simulink model "QBOT_follower1"  (R2022b)
settings: Solver=ode1  StartTime=0.0  StopTime=inf  FixedStep=Ts  RelTol=1e-3  EnableMultiTasking=on
model workspace (MAT data in the model file):
  Sig = Simulink.Signal
  Sig.DataType = 'auto'
  Sig.Dimensions = -1
  Sig.DimensionsMode = 'auto'
  Sig.Complexity = 'auto'
  Sig.SampleTime = -1
  Sig.SamplingMode = 'auto'
  downCamStepSize = Simulink.Parameter
  downCamStepSize.Value = Simulink.data.Expression
  downCamStepSize.Value.ExpressionString = "qc_get_step_size*ceil(1/60/qc_get_step_size)"
  downCamStepSize.DataType = 'auto'
  downCamStepSize.Complexity = 'real'
  downCamStepSize.Dimensions = -1
  lidarStepSize = Simulink.Parameter
  lidarStepSize.Value = Simulink.data.Expression
  lidarStepSize.Value.ExpressionString = "qc_get_step_size*ceil(1/5/qc_get_step_size)"
  lidarStepSize.DataType = 'auto'
  lidarStepSize.Complexity = 'real'
  lidarStepSize.Dimensions = -1
  mainStepSize = Simulink.Parameter
  mainStepSize.Value = Simulink.data.Expression
  mainStepSize.Value.ExpressionString = "qc_get_step_size"
  mainStepSize.DataType = 'auto'
  mainStepSize.Complexity = 'real'
  mainStepSize.Dimensions = -1
  mode = Simulink.Parameter
  mode.Value = 2
  mode.Description = '0 - education speeds via wheel speed commands
    | 1 - education speeds via body speed commands
    | 2 - research speeds via wheel speed commands
    | 3 - research speeds via body speed commands'
  mode.DataType = 'auto'
  mode.Complexity = 'real'
  mode.Dimensions = [1 1]
  realSenseStepSize = Simulink.Parameter
  realSenseStepSize.Value = Simulink.data.Expression
  realSenseStepSize.Value.ExpressionString = "qc_get_step_size*ceil(1/30/qc_get_step_size)"
  realSenseStepSize.DataType = 'auto'
  realSenseStepSize.Complexity = 'real'
  realSenseStepSize.Dimensions = -1
values from neighbouring files (symbols this model uses):
  b = 0.17    [follower_1_parameters.m]    (also in follower_2_parameters.m; leader_parameters.m)
  d = 0.393    [follower_1_parameters.m]    (also in follower_2_parameters.m; leader_parameters.m)
  d_safe = 0.75    [follower_1_parameters.m]    (also in follower_2_parameters.m = 0.8)
  delay1 = 4    [follower_1_parameters.m]
  parameters = [r d wrlmax Ts b]    [follower_1_parameters.m]    (also in follower_2_parameters.m; leader_parameters.m)
  Q_k = [Q_k Qi]    [follower_1_parameters.m]    (also in follower_2_parameters.m; leader_parameters.m)
  R = 0*eye(2)    [follower_1_parameters.m]    (also in follower_2_parameters.m; leader_parameters.m)
  r = 0.04445    [follower_1_parameters.m]    (also in follower_2_parameters.m; leader_parameters.m)
  R_d = 0*eye(2)    [follower_1_parameters.m]    (also in follower_2_parameters.m; leader_parameters.m)
  T = [[r/2 r/2];[r/d -r/d]]    [follower_1_parameters.m]    (also in follower_2_parameters.m; leader_parameters.m)
  Ts = 1/60    (= 0.0166666666667)    [follower_1_parameters.m]    (also in follower_2_parameters.m; leader_parameters.m)
  u_pre = [0;0]    [follower_1_parameters.m]    (also in follower_2_parameters.m; leader_parameters.m)
  X0 = [vicon_data(1); vicon_data(2); vicon_data(6)]    [follower_1_parameters.m]    (also in follower_2_parameters.m; leader_parameters.m)
libraries: quarc_library x13, simulink x5, spsDiscreteVariableTimeDelayLib x1, dspsigops x1
settings Model: SimulationMode=external  ExtModeTrigDuration=10000  Creator=mbohra  LastModifiedBy=user
settings SolverCC: AlgebraicLoopSolver=TrustRegion  PositivePriorityOrder=on
settings DataIOCC: ReturnWorkspaceOutputs=off
settings OptimizationCC: ReuseModelBlockBuffer=on
settings DebuggingCC: UnconnectedInputMsg=warning  UnconnectedOutputMsg=warning  UnconnectedLineMsg=warning  ArithmeticOperatorsInVariantConditions=warning
settings HardwareCC: ProdBitPerLong=64  ProdLargestAtomicInteger=LongLong  ProdLargestAtomicFloat=Double  ProdLongLongMode=on  ProdHWDeviceType=ARM Compatible->ARM 64-bit (LP64)
settings ModelReferenceCC: EnableRefExpFcnMdlSchedulingChecks=on
settings SFSimCC: SimUseLocalCustomCode=off  CustomCodeUndefinedFunction=UseInterfaceOnly
settings RTWCC: Description=QUARC Linux QBot Platform Target Using Toolchain  SystemTargetFile=quarc_linux_qbot_platform.tlc  TemplateMakefile=quarc_default_tmf  RTWUseLocalCustomCode=off  Toolchain=QUARC linux_qbot_platform | gmake (64-bit Windows)  BuildConfiguration=Faster Runs
settings CodeAppCC: StateflowObjectComments=on
settings STFCustomTargetCC: TargetLangStandard=C99 (ISO)  ConcurrentExecutionCompliant=on  GRTInterface=on  UseToolchainInfoCompliant=on  SystemTargetFile=quarc_linux_qbot_platform.tlc
settings GRTTargetCC: ParMdlRefBuildCompliant=off  CompOptLevelCompliant=off  CombineOutputUpdateFcns=off  MatFileLogging=off  CPPClassGenCompliant=off  GRTInterface=on  ExtMode=on  ExtModeMexFile=quarc_comm  ExtModeMexArgs='-w -d /tmp -uri %u','tcpip://192.168.0.130:17001'
settings ConfigComp: CovMetricSettings=dswe

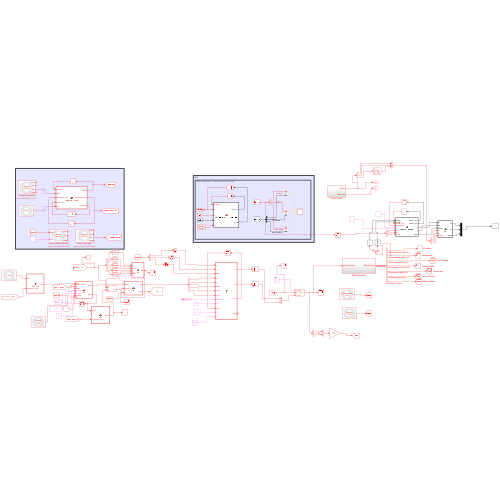
[thumbnail: Simulink's stored preview of the top-level diagram]
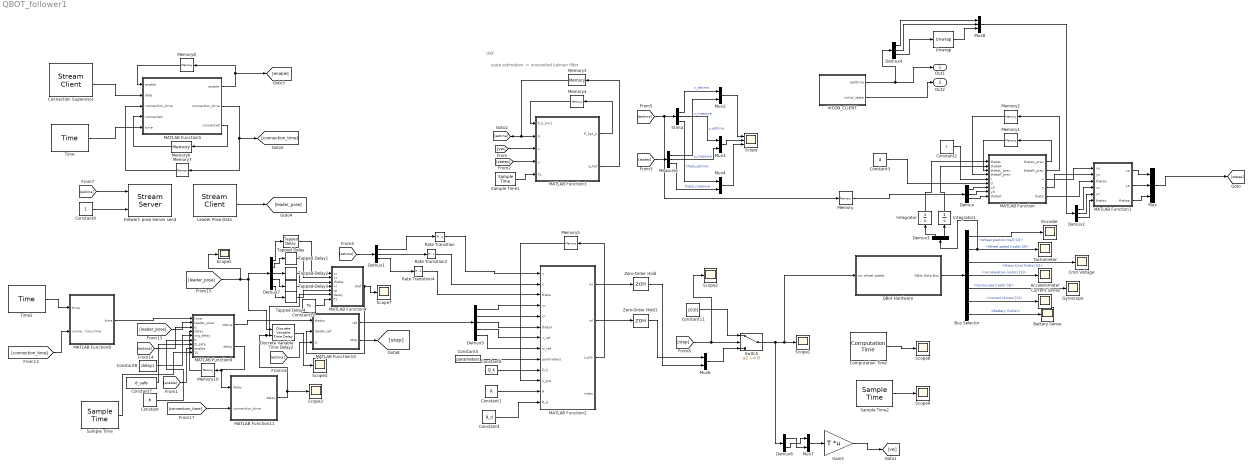
== system QBOT_follower1 ==
  note: UKF
  note: state estimation -> unscented kalman filter
  Accelerometer : Scope
  Battery Sense : Scope
  Bus Selector : BusSelector  OutputSignals=Wheel position (rad) [2],Wheel speed (rad/s) [2],Motor Cmd (Volts) [2],Acceleration (m/s/s) [3],Gyroscope (rad/s) [3],Current (Amps) [2],Battery (Volts)
  Cmd Voltage : Scope
  Computation Time : quarc_library/Sources/Time/Computation Time  sample_time=qc_get_step_size  use_model=on  use_cpu_time=off
  Connection Supervisor : quarc_library/Communications/Basic/Stream Client  uri_source=Specify via dialog (do not evaluate)  uri=tcpip://192.168.0.5:18013  send_buffer_size=1460  receive_buffer_size=1460  byte_order=little endian (Intel - LSB first)  optimization=Minimum latency  send_options=Do not send data  receive_options=Receive all data  default_value=[0]  sample_time=-1  active=off  implementation=Use blocking I/O in a separate thread  send_fifo_size=1000  receive_fifo_size=1000  send_priority=0  receive_priority=0  send_dimensions=off  receive_dimensions=off  max_dimensions=-1  data_type=Inherited via back propagation  type_expr=BusObject
      settings: AttributesFormatString="\"tcpip://192.168.0.5:18013\""
  Constant : Constant  Value=b
  Constant1 : Constant  Value=R
  Constant10 : Constant  Value=Ts
  Constant11 : Constant  Value=[0;0]  VectorParams1D=off
  Constant2 : Constant  Value=r
  Constant3 : Constant  Value=d
  Constant4 : Constant  Value=R_d
  Constant5 : Constant  Value=parameters
  Constant6 : Constant  Value=Q_k
  Constant7 : Constant  Value=d_safe
  Constant8 : Constant  Value=delay1
  Constant9 : Constant
  Current Sense : Scope
  Demux{,1..2,4} (4 alike) : Demux  Outputs=3
  Demux3 : Demux  Outputs=2
  Demux5 : Demux  Outputs=5
  Demux6 : Demux  Outputs=2
  Demux7 : Demux  Outputs=5
  Discrete Variable Time Delay2 : spsDiscreteVariableTimeDelayLib/Discrete Variable Time Delay  MaxDelay=60  InitialValue=0  Ts=Ts  DFT=on
      settings: LibrarySourceBlock=|
      | sps_lib/Control/Discrete Variable
      | Time Delay
  Encoder : Scope
  Follwer1 pose Server send : quarc_library/Communications/Basic/Stream Server  uri_source=Specify via dialog (do not evaluate)  uri=tcpip://192.168.0.130:18012  send_buffer_size=1460  receive_buffer_size=1460  byte_order=little endian (Intel - LSB first)  optimization=Minimum latency  send_options=Send all data  receive_options=Do not receive data  default_value=[0]  sample_time=-1  active=off  implementation=Use blocking I/O in a separate thread  send_fifo_size=1000  receive_fifo_size=1000  send_priority=0  receive_priority=0  send_dimensions=off  receive_dimensions=off  max_dimensions=-1  data_type=Inherited via back propagation  type_expr=BusObject
      settings: AttributesFormatString="\"tcpip://192.168.0.130:18012\""
  Gain5 : Gain  Gain=T  Multiplication=Matrix(K*u)
  Gyroscope : Scope
  Integrator : Integrator
  Integrator1 : Integrator
  Leader Pose Data : quarc_library/Communications/Basic/Stream Client  uri_source=Specify via dialog (do not evaluate)  uri=tcpip://192.168.0.230:18010  send_buffer_size=1460  receive_buffer_size=1460  byte_order=little endian (Intel - LSB first)  optimization=Minimum latency  send_options=Do not send data  receive_options=Receive all data  default_value=[0;0;0;0;0]  sample_time=-1  active=off  implementation=Use blocking I/O in a separate thread  send_fifo_size=1000  receive_fifo_size=1000  send_priority=0  receive_priority=0  send_dimensions=off  receive_dimensions=off  max_dimensions=-1  data_type=Inherited via back propagation  type_expr=BusObject
      settings: AttributesFormatString="\"tcpip://192.168.0.230:18010\""
  MATLAB Function : MATLAB Function  TreatAsAtomicUnit=on
  MATLAB Function1 : MATLAB Function  TreatAsAtomicUnit=on
  MATLAB Function10 : MATLAB Function  TreatAsAtomicUnit=on
  MATLAB Function11 : MATLAB Function  TreatAsAtomicUnit=on
  MATLAB Function2 : MATLAB Function  TreatAsAtomicUnit=on
  MATLAB Function3 : MATLAB Function  TreatAsAtomicUnit=on
  MATLAB Function4 : MATLAB Function  TreatAsAtomicUnit=on
  MATLAB Function5 : MATLAB Function  TreatAsAtomicUnit=on
  MATLAB Function8 : MATLAB Function  TreatAsAtomicUnit=on
  MATLAB Function9 : MATLAB Function  TreatAsAtomicUnit=on
  Measures : Demux  Outputs=3
  Memory : Memory  InitialCondition=X0
  Memory{1..2,6..8} (5 alike) : Memory
  Memory10 : Memory  InitialCondition=delay1
  Memory3 : Memory  InitialCondition=X0  InheritSampleTime=on
  Memory4 : Memory  InitialCondition=1e-6*eye(3)  InheritSampleTime=on
  Memory5 : Memory  InitialCondition=u_pre
  Mux : Mux  Inputs=3
  Mux{2..4,6..7} (5 alike) : Mux  Inputs=2
  Mux8 : Mux  Inputs=3
  QBot Hardware : Subsystem
  Rate Transition : RateTransition  OutPortSampleTime=Ts
  Rate Transition2 : RateTransition  OutPortSampleTime=Ts
  Rate Transition4 : RateTransition  OutPortSampleTime=Ts
  Sample Time : quarc_library/Sources/Time/Sample Time  Priority=-99  sample_time=qc_get_step_size
  Sample Time1 : quarc_library/Sources/Time/Sample Time  Priority=-99  sample_time=Ts
  Sample Time2 : quarc_library/Sources/Time/Sample Time  Priority=-99  sample_time=qc_get_step_size
  Scope : Scope  NumInputPorts=3
  Scope{1..8} (8 alike) : Scope
  Stima : Demux  Outputs=3
  Switch : Switch  Criteria=u2 ~= 0  SaturateOnIntegerOverflow=off  InputSameDT=off
  Tachometer : Scope
  Tapped Delay{,1..4} (5 alike) : simulink/Discrete/Tapped Delay  vinit=0.0  samptime=Ts  NumDelays=1500  DelayOrder=Newest  includeCurrent=on
  Time : quarc_library/Sources/Time/Time  time_source=Wall clock  sample_time=qc_get_step_size
  Time2 : quarc_library/Sources/Time/Time  time_source=Wall clock  sample_time=qc_get_step_size
  Unwrap : dspsigops/Unwrap  tol=pi  InputProcessing=Columns as channels (frame based)  running=off
  VICON_CLIENT : Subsystem
  Zero-Order Hold : ZeroOrderHold  SampleTime=Ts
  Zero-Order Hold1 : ZeroOrderHold  SampleTime=Ts
  Out1 : Outport
  Out2 : Outport  Port=2
  wires:
  QBot Hardware/1(QBot Data Bus) -> Bus Selector/1
  Bus Selector/1 -> Encoder/1  "<Wheel position (rad) [2]>"
  Bus Selector/3 -> Cmd Voltage/1  "<Motor Cmd (Volts) [2]>"
  Bus Selector/4 -> Accelerometer/1  "<Acceleration (m/s/s) [3]>"
  Bus Selector/6 -> Current Sense/1  "<Current (Amps) [2]>"
  Bus Selector/2 -> Demux3/1, Tachometer/1  "<Wheel speed (rad/s) [2]>"
  Bus Selector/5 -> Gyroscope/1  "<Gyroscope (rad/s) [3]>"
  Bus Selector/7 -> Battery Sense/1  "<Battery (Volts)>"
  VICON_CLIENT/1(realtime) -> Demux4/1, Out1/1
  VICON_CLIENT/2(initial_state) -> Out2/1
  MATLAB Function/3(x) -> MATLAB Function1/1(xo)
  MATLAB Function/4(y) -> MATLAB Function1/2(yo)
  MATLAB Function/5(theta) -> MATLAB Function1/3(thetao)
  Demux2/1 -> MATLAB Function1/4(xv)
  Demux2/2 -> MATLAB Function1/5(yv)
  Demux2/3 -> MATLAB Function1/6(thetav)
  MATLAB Function1/1(xa) -> Mux/1
  MATLAB Function1/2(ya) -> Mux/2
  MATLAB Function1/3(thetaa) -> Mux/3
  Mux/1 -> [states]
  Stima/1 -> Mux2/1  "x_estima"
  Sample Time1/1 -> MATLAB Function3/5(Ts)
  Measures/2 -> Mux3/2  "y_measure"
  Memory4/1 -> MATLAB Function3/1(P_k_km1)
  Measures/1 -> Mux2/2  "x_measure"
  Mux2/1 -> Scope/1
  [vw] -> MATLAB Function3/3(u)
  Mux3/1 -> Scope/2
  [states] -> Measures/1
  Stima/2 -> Mux3/1  "y_estima"
  Measures/3 -> Mux4/2  "theta_measure"
  [states] -> MATLAB Function3/4(y)
  [estima] -> Memory/1, Stima/1
  MATLAB Function3/2(q_hat) -> Memory3/1
  Memory3/1 -> MATLAB Function3/2(q), [estima]
  Mux4/1 -> Scope/3
  MATLAB Function3/1(P_kp1_k) -> Memory4/1
  Stima/3 -> Mux4/1  "theta_estima"
  Constant3/1 -> MATLAB Function/6(d)
  Demux3/1 -> Integrator/1
  Demux3/2 -> Integrator1/1
  Integrator/1 -> MATLAB Function/1(thetaL)
  Integrator1/1 -> MATLAB Function/2(thetaR)
  Demux/3 -> MATLAB Function/9(theta0)
  Demux/1 -> MATLAB Function/7(x0)
  Demux/2 -> MATLAB Function/8(y0)
  Memory/1 -> Demux/1
  Constant2/1 -> MATLAB Function/5(r)
  MATLAB Function/1(thetaL_prev) -> Memory1/1
  MATLAB Function/2(thetaR_prev) -> Memory2/1
  Memory1/1 -> MATLAB Function/3("thetaL_prev ")
  Memory2/1 -> MATLAB Function/4("thetaR_prev ")
  Demux1/2 -> Rate Transition2/1
  Demux1/1 -> Rate Transition/1
  Rate Transition4/1 -> MATLAB Function2/3(theta)
  Constant6/1 -> MATLAB Function2/10(Q_k)
  Zero-Order Hold/1 -> Mux6/2
  MATLAB Function2/2(wl) -> Zero-Order Hold1/1
  Memory5/1 -> MATLAB Function2/11("u_pre ")
  Demux1/3 -> Rate Transition4/1
  Rate Transition/1 -> MATLAB Function2/1(x)
  Rate Transition2/1 -> MATLAB Function2/2(y)
  MATLAB Function2/1(wr) -> Zero-Order Hold/1
  Constant5/1 -> MATLAB Function2/9(parameters)
  MATLAB Function2/3(u_pre) -> Memory5/1
  Zero-Order Hold1/1 -> Mux6/1
  Constant4/1 -> MATLAB Function2/13(R_d)
  [estima] -> Demux1/1
  Constant1/1 -> MATLAB Function2/12(R)
  Gain5/1 -> [vw]
  Demux4/3 -> Unwrap/1
  Unwrap/1 -> Mux8/3
  Demux4/1 -> Mux8/1
  Demux4/2 -> Mux8/2
  Mux8/1 -> Demux2/1
  Demux5/1 -> MATLAB Function2/4(xr)
  Demux5/2 -> MATLAB Function2/5(yr)
  Demux5/3 -> MATLAB Function2/6(thetar)
  Demux5/4 -> MATLAB Function2/7(v_ref)
  Demux5/5 -> MATLAB Function2/8(w_ref)
  Constant11/1 -> Switch/1
  [stop] -> Scope2/1, Switch/2
  Mux6/1 -> Switch/3
  Switch/1 -> Demux6/1, QBot Hardware/1(rsc wheel speed), Scope1/1
  Demux6/1 -> Mux7/2
  Demux6/2 -> Mux7/1
  Mux7/1 -> Gain5/1
  Connection Supervisor/3 -> MATLAB Function5/2(data)
  MATLAB Function5/1(enable) -> Memory8/1, [enable]
  [estima] -> Follwer1 pose Server send/1
  Leader Pose Data/3 -> [leader_pose]
  MATLAB Function5/3(connected) -> Memory6/1
  Memory6/1 -> MATLAB Function5/4("connected ")
  Time/1 -> MATLAB Function5/5(time)
  MATLAB Function5/2(connection_time) -> Memory7/1, [connection_time]
  Memory7/1 -> MATLAB Function5/3("connection_time ")
  Memory8/1 -> MATLAB Function5/1("enable ")
  Time2/1 -> MATLAB Function8/1("time ")
  [connection_time] -> MATLAB Function8/2(connection_time)
  [leader_pose] -> MATLAB Function9/2(leader_pose)
  MATLAB Function8/1(time) -> MATLAB Function9/1(time)
  [estima] -> MATLAB Function9/3(q)
  MATLAB Function9/2(delay) -> MATLAB Function11/1("delay "), Memory10/1
  Memory10/1 -> MATLAB Function9/4("delay ")
  Constant8/1 -> MATLAB Function9/5(org_delay)
  MATLAB Function9/1(status) -> MATLAB Function10/1(status)
  Discrete Variable Time Delay2/1 -> Scope4/1
  [leader_pose] -> Scope5/1, Demux7/1, Discrete Variable Time Delay2/1
  [estima] -> MATLAB Function10/3(q)
  [connection_time] -> MATLAB Function11/2(connection_time)
  MATLAB Function11/1(delay) -> Scope3/1, MATLAB Function4/6(delay), Discrete Variable Time Delay2/2
  MATLAB Function10/1(ref) -> Demux5/1
  MATLAB Function10/2(stop) -> [stop]
  Constant/1 -> MATLAB Function9/6(b)
  Constant7/1 -> MATLAB Function9/7(D_safe)
  Constant9/1 -> Follwer1 pose Server send/2
  [enable] -> MATLAB Function9/8(enable)
  Sample Time/1 -> MATLAB Function9/9(Ts)
  Sample Time2/1 -> Scope6/1
  Demux7/4 -> Tapped Delay3/1
  Tapped Delay3/1 -> MATLAB Function4/4(vr)
  Tapped Delay1/1 -> MATLAB Function4/2(yr)
  Tapped Delay4/1 -> MATLAB Function4/5(wr)
  Tapped Delay/1 -> MATLAB Function4/1(xr)
  Tapped Delay2/1 -> MATLAB Function4/3(thetar)
  Demux7/1 -> Tapped Delay/1
  Demux7/5 -> Tapped Delay4/1
  Demux7/3 -> Tapped Delay2/1
  Demux7/2 -> Tapped Delay1/1
  Constant10/1 -> MATLAB Function4/7(Ts)
  MATLAB Function4/1(dref) -> MATLAB Function10/2(leader_ref), Scope7/1
  Computation Time/1 -> Scope8/1

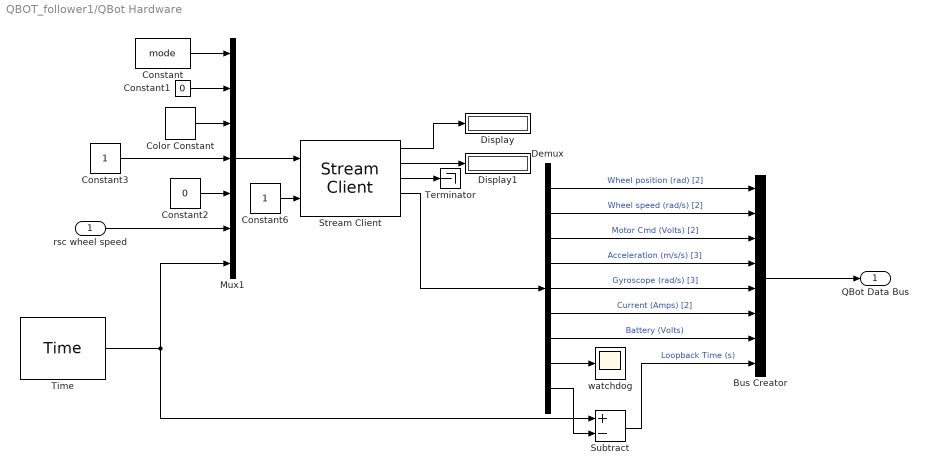
== system QBOT_follower1/QBot Hardware ==
  rsc wheel speed : Inport
  Bus Creator : BusCreator  Inputs=8
  Color Constant : quarc_library/Sources/Signals/Color Constant  color=[0 1 1]
      settings: SourceProductName=QUARC Targets
  Constant : Constant  Value=mode
  Constant1 : Constant  Value=0
  Constant2 : Constant  Value=0
  Constant3 : Constant
  Constant6 : Constant
  Demux : Demux  Outputs=[2 2 2 3 3 2 1 1 1]
  Display : Display
  Display1 : Display
  Mux1 : Mux  Inputs=7
  Stream Client : quarc_library/Communications/Basic/Stream Client  uri_source=Specify via dialog (do not evaluate)  uri=tcpip://localhost:18888  send_buffer_size=1460  receive_buffer_size=1460  byte_order=little endian (Intel - LSB first)  optimization=Minimum latency  send_options=Send most recent data  receive_options=Receive most recent data  default_value=zeros(17,1)  sample_time=qc_get_step_size  active=off  implementation=Use blocking I/O in a separate thread  send_fifo_size=1000  receive_fifo_size=1000  send_priority=0  receive_priority=0  send_dimensions=off  receive_dimensions=off  max_dimensions=-1  data_type=Inherited via back propagation  type_expr=BusObject
      settings: AttributesFormatString="\"tcpip://localhost:18888\""
  Subtract : Sum  Inputs=+-
  Terminator : Terminator
  Time : quarc_library/Sources/Time/Time  time_source=Wall clock  sample_time=qc_get_step_size
  watchdog : Scope
  QBot Data Bus : Outport
  wires:
  Demux/2 -> Bus Creator/2  "Wheel speed (rad/s) [2]"
  Constant/1 -> Mux1/1
  Stream Client/3 -> Terminator/1
  Stream Client/1 -> Display/1
  Constant6/1 -> Stream Client/2
  Stream Client/2 -> Display1/1
  Color Constant/1 -> Mux1/3
  Constant1/1 -> Mux1/2
  Demux/3 -> Bus Creator/3  "Motor Cmd (Volts) [2]"
  Mux1/1 -> Stream Client/1
  Stream Client/4 -> Demux/1
  Demux/1 -> Bus Creator/1  "Wheel position (rad) [2]"
  Demux/7 -> Bus Creator/7  "Battery (Volts)"
  Demux/5 -> Bus Creator/5  "Gyroscope (rad/s) [3]"
  Demux/6 -> Bus Creator/6  "Current (Amps) [2]"
  Demux/9 -> Subtract/2
  Constant2/1 -> Mux1/5
  Demux/4 -> Bus Creator/4  "Acceleration (m/s/s) [3]"
  Time/1 -> Subtract/1, Mux1/7
  Bus Creator/1 -> QBot Data Bus/1
  Subtract/1 -> Bus Creator/8  "Loopback Time (s)"
  Demux/8 -> watchdog/1
  Constant3/1 -> Mux1/4
  rsc wheel speed/1 -> Mux1/6

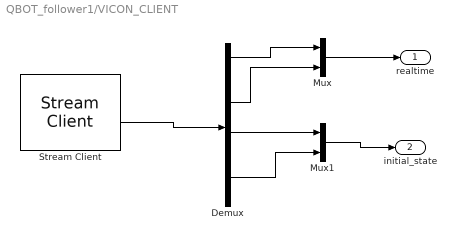
== system QBOT_follower1/VICON_CLIENT ==
  Demux : Demux  Outputs=[2 1 2 1 1 2 1 2 1 1]
  Mux : Mux  Inputs=2
  Mux1 : Mux  Inputs=2
  Stream Client : quarc_library/Communications/Basic/Stream Client  uri_source=Specify via dialog (do not evaluate)  uri=tcpip://192.168.0.5:18099  send_buffer_size=1460  receive_buffer_size=1460  byte_order=little endian (Intel - LSB first)  optimization=Minimum latency  send_options=Do not send data  receive_options=Receive most recent data  default_value=zeros(1,14)  sample_time=-1  active=off  implementation=Use blocking I/O in a separate thread  send_fifo_size=1000  receive_fifo_size=1000  send_priority=0  receive_priority=0  send_dimensions=off  receive_dimensions=off  max_dimensions=-1  data_type=Inherited via back propagation  type_expr=BusObject
      settings: AttributesFormatString="\"tcpip://192.168.0.5:18099\""
  realtime : Outport
  initial_state : Outport  Port=2
  wires:
  Stream Client/3 -> Demux/1
  Demux/9 -> Mux1/2
  Demux/4 -> Mux/2
  Demux/6 -> Mux1/1
  Demux/1 -> Mux/1
  Mux1/1 -> initial_state/1
  Mux/1 -> realtime/1

== matlab function QBOT_follower1/MATLAB Function8 ==
  data: time input; time output; connection_time input
function time = time_chn(time, connection_time)

time = time - connection_time

== matlab function QBOT_follower1/MATLAB Function9 ==
  data: status output; time input; delay output; leader_pose input; q input; delay input; org_delay input; b input; D_safe input; enable input; Ts input
function [status,delay]= fcn(time, leader_pose, q, delay, org_delay,b, D_safe, enable,Ts)

leader_B=[leader_pose(1)+b*cos(leader_pose(3));leader_pose(2)+b*sin(leader_pose(3))];
follower1_B=[q(1)+b*cos(q(3));q(2)+b*sin(q(3))];

% leader_B=[leader_pose(1);leader_pose(2)];
% follower1_B=[q(1);q(2)];


%stop = 1, Go = 0
if time<delay
    status = 1;
else
   
    if check_intersection(leader_B,follower1_B,D_safe)
        status = 1;
        delay = delay+Ts;
    else
        if delay>org_delay
            delay = delay-Ts;
        end
        status = 0;
    end
end

if enable == 0
    status = 1;
end

end

function collision = check_intersection(z1,z2,d_safe)
if  norm(z1-z2,2)<d_safe %||  norm(z1-z2,2)<r1+r2
    collision=1;
else
    collision=0;
end

end

== matlab function QBOT_follower1/MATLAB Function10 ==
  data: status input; ref output; leader_ref input; q input; stop output
function [ref, stop]= fcn(status,leader_ref, q)

if status == 1
    stop =1;
    ref = [q;0;0];
else
    stop =0;
    ref = leader_ref;
end

== matlab function QBOT_follower1/MATLAB Function2 ==
  data: x input; wr output; y input; theta input; xr input; yr input; wl output; thetar input; v_ref input; w_ref input; parameters input; Q_k input; u_pre input; u_pre output; R input; R_d input; index output
function [wr, wl, u_pre,index] = fcn(x,y,theta,xr,yr,thetar,v_ref,w_ref, parameters, Q_k,u_pre, R,R_d)

r=parameters(1);        % radius od wheels [m]
d=parameters(2);      % distance between the two wheels [m]
wrlmax=parameters(3);   % max angular velocity [rad/s] 
Ts=parameters(4);      % sampling time [s]
b=parameters(5);         % distance point b [m]


T=[[r/2 r/2];[r/d -r/d]];
T_inv=inv(T);
Hd=[-1/wrlmax 0 ; 0 -1/wrlmax ; 1/wrlmax 0 ; 0 1/wrlmax];


A = eye(2);
Bu = eye(2)*Ts;
Bd = eye(2)*Ts;


z_curr=[x+b*cos(theta)-(xr+b*cos(thetar));
        y+b*sin(theta)-(yr+b*sin(thetar))];
    
    
    
    T_FL = [cos(theta) sin(theta); -sin(theta)/b cos(theta)/b];
    T_FL_inv=inv(T_FL);
    
    %Compute current input constraint set
    %     U_curr=T_FL_inv*U_uni;
    
    H_curr=Hd*T_inv*T_FL;
    g=ones(4,1);
    % U_curr=Polyhedron(H_curr,g);
    


    Qpre=Q_k(1:2,1:2); %DOUBLE CHECK%%%%%%%%%%%%%%%%%%%%%%%%%%%%%%%%%%%%%%%%
    index=inf;

    isintern=0;
    for j=1:2:length(Q_k)
        Q_curr=Q_k(1:2,j:j+1);
        if  z_curr'*inv(Q_curr)*z_curr<=1
            
            index=(j-1)/2+1;
            isintern=1;
            if index>1
                Qpre=Q_k(1:2,j-2:j-1);
            end
            break
        end
    end
    
    
    
    if isintern==0
        error('The current point is outside the domain of attraction of the algorithm')
    end
    
    
    
    T_FL_r=[cos(thetar) sin(thetar); -sin(thetar)/b cos(thetar)/b];
    ur=inv(T_FL_r)*[v_ref;w_ref];
   

    
    if index>1
        
  
        ukhat = online_phase_CDC(z_curr,Qpre,A,Bu,H_curr,g,R_d,ur,u_pre);
     
        
       
    else
        
        ukhat=-inv(Bd)*z_curr;
        
        ur=online_terminal_optim_QP(ur,ukhat,H_curr,g);

    end
    
    
    uk=ukhat+ur;
    u_pre=ukhat;
    
 
    
    
    
    vw=T_FL*uk;
    
    wrwl=T_inv*vw;


    wr=wrwl(1);
    wl=wrwl(2);




end





function uk = online_phase_CDC(x_curr,Qpre,A,B,H,g,Rd,ur,u_pre)



%Set theoretic MPC online optimization
obj_fun=@(u)(A*x_curr+B*(u+ur)-B*ur)'*(A*x_curr+B*(u+ur)-B*ur)+(u-u_pre)'*Rd*(u-u_pre);


    function [c,ceq]=quad_constr(u,H,g,Qpre,ur,A,B,x_curr)
        c1=H*(u+ur)-g;
        c2=(A*x_curr+B*(u+ur)-B*ur)'*inv(Qpre)*(A*x_curr+B*(u+ur)-B*ur)-1;
        c=[c1;c2];
        ceq=[];
    end



options=optimoptions('fmincon','Display','off','Algorithm','sqp');
usol = fmincon(obj_fun,[0;0],[],[],[],[],[],[],@(u)quad_constr(u,H,g,Qpre,ur,A,B,x_curr),options);
uk=usol;


test_g=H*(uk+ur)-g;

test1=test_g(1);
test2=test_g(2);
test3=test_g(3);
test4=test_g(4);

test5=(A*x_curr+B*(uk))'*inv(Qpre)*(A*x_curr+B*(uk))-1;


test=test1<0 & test2<0 & test3<0 &test4<0 & test5<0;


obj_fun=(A*x_curr+B*(uk+ur)-B*ur)'*(A*x_curr+B*(uk+ur)-B*ur)+(uk-u_pre)'*Rd*(uk-u_pre);




% if test~=1
% 
%     error('ATTENZIONE')
% 
% end



end




function ur_hat = online_terminal_optim_QP(ur,u0,H,g)


H_obj=eye(2);
f_obj=-ur;
A_constr=H;
b_constr=g-H*u0;


options = optimoptions(@quadprog,'Algorithm','active-set','Display','off');


usol=quadprog(H_obj,f_obj,A_constr,b_constr,[],[],[],[],[0;0],options);
ur_hat=usol;

end

== matlab function QBOT_follower1/MATLAB Function11 ==
  data: delay input; connection_time input; delay output
function delay = fcn(delay,connection_time)

delay = delay; %+ connection_time;

end

== matlab function QBOT_follower1/MATLAB Function1 ==
  data: xo input; xa output; yo input; thetao input; xv input; yv input; thetav input; ya output; thetaa output
function [xa,ya,thetaa] = fcn(xo,yo,thetao,xv,yv,thetav)
% a - average
% v- vicon_data
% o - odometry
 mo = 5;
 mv = 95;

xa = (mo*xo+mv*xv)/100;
ya = (mo*yo+mv*yv)/100;
thetaa = (mo*thetao+mv*thetav)/100;

== matlab function QBOT_follower1/MATLAB Function ==
  data: thetaL_prev output; thetaR_prev output; x output; thetaL input; y output; thetaR input; thetaL_prev input; thetaR_prev input; r input; d input; x0 input; y0 input; theta0 input; theta output
function [thetaL_prev, thetaR_prev,x,y,theta]=computeOdometry(thetaL,thetaR,thetaL_prev, thetaR_prev,r,d,x0,y0,theta0)
    delta_sL=r*(thetaL - thetaL_prev);
    delta_sR=r*(thetaR - thetaR_prev);
    delta_theta=(delta_sR-delta_sL)/d;
    delta_s=(delta_sR+delta_sL)/2;
    theta=theta0+delta_theta/2;
    x=x0+delta_s*cos(theta);
    y=y0+delta_s*sin(theta); 
    thetaL_prev = thetaL;
    thetaR_prev = thetaR;
end

== matlab function QBOT_follower1/MATLAB Function4 ==
  data: xr input; yr input; thetar input; vr input; wr input; dref output; delay input; Ts input
function dref = fcn(xr, yr, thetar, vr, wr, delay,Ts)
n = delay/Ts;
xrn = xr(n+1);
yrn = yr(n+1);
thetarn = thetar(n+1);
vrn = vr(n+1);
wrn = wr(n+1);
dref= [xrn;yrn;thetarn; vrn; wrn];
end

== matlab function QBOT_follower1/MATLAB Function5 ==
  data: enable input; data input; enable output; connection_time input; connection_time output; connected input; connected output; time input
function [enable,connection_time,connected] = resetconnection( enable,data,connection_time,connected, time)


if connected == 0
    connection_time = time;
    if data ==1
        connected = 1;
        enable = 1 ;
    end
end

== matlab function QBOT_follower1/MATLAB Function3 ==
  data: P_k_km1 input; P_kp1_k output; q input; u input; q_hat output; y input; Ts input
function [P_kp1_k,q_hat]= my_unscented_kalman_filter(P_k_km1,q,u,y,Ts)
Q=1e-6*eye(3);
R=1e-4*eye(3);
alpha=0.9; beta=2; kappa=0;
%Calculate the Sigma points
M=3;
c=alpha^2*(M+kappa);
q_hat_i=zeros(M,2*M+1);
q_hat_i(:,1)=q;
Delta_x=real(sqrtm(c*P_k_km1));
for i=1:M
    q_hat_i(:,i+1)=q+Delta_x(:,i);
    q_hat_i(:,i+1+M)=q-Delta_x(:,i);
end
%Output of the sigma points
y_hat_i=q_hat_i(1:3,:);
%predicted measurement at time k
W_M=zeros(1,2*M+1);
W_M(1)=1-(M/(alpha^2*(M+kappa)));
W_M(2:2*M+1)=(1/(2*alpha^2*(M+kappa)));
y_k=zeros(3,1);
for i=1:2*M+1
    y_k=y_k+W_M(i)*y_hat_i(:,i);
end
%Estimate of the covariance of predicted measurement
W_c=zeros(1,2*M+1);
W_c(1)=(2-alpha^2+beta)-(M/(alpha^2*(M+kappa)));
W_c(2:2*M+1)=(1/(2*alpha^2*(M+kappa)));
P_y=zeros(3,3);
for i=1:2*M+1
    P_y=P_y+W_c(i)*(y_hat_i(:,i)-y_k)*(y_hat_i(:,i)-y_k)'+R;
end
%%Estimate of the cross-covariance between predicted x and y
P_xy=zeros(M,3);
for i=1:2*M+1
    P_xy=P_xy+(1/(2*alpha^2*(M+kappa)))*(q_hat_i(:,i)-q)*(y_hat_i(:,i)-y_k)';
end
%Kalman gain
K=P_xy/(P_y);
q_k_k = q+K*(y-y_k);
P_k_k = P_k_km1 -K*P_y*K';
% State prediction and state estimation error covariance
q_hat_i_k_k=zeros(M,2*M+1);
q_hat_i_k_k(:,1)=q_k_k;
Delta_x=real(sqrtm(c*P_k_k));
for i=1:M
    q_hat_i_k_k(:,i+1)=q_k_k+Delta_x(:,i);
    q_hat_i_k_k(:,i+1+M)=q_k_k-Delta_x(:,i);
end
%Predicted state for each sigma point
q_hat_kp1_k=zeros(M,2*M+1);
for i=1:2*M+1
    q_hat_kp1_k(:,i)=q_hat_i_k_k(:,i)+Ts*[cos(q_hat_i_k_k(3,i)) 0;
        sin(q_hat_i_k_k(3,i)) 0;
        0          1]*u;
end
%Predicted state k+1 at time k
q_hat=zeros(M,1);
for i=1:2*M+1
    q_hat=q_hat + W_M(i)*q_hat_kp1_k(:,i);
end
%Covariance of the predicted state
P_kp1_k=zeros(M,M);
for i=1:2*M+1
    P_kp1_k=P_kp1_k+W_c(i)*(q_hat_kp1_k(:,i)-q_hat)*(q_hat_kp1_k(:,i)-q_hat)'+Q;
end
end
